simulink model "Drone_BBall_Developer"  (R2020a)
settings: Solver=FixedStepAuto  StartTime=0.0  StopTime=60  FixedStep=.001  RelTol=1e-3
values from neighbouring files (symbols this model uses):
  b = .25*m    (= 0.25)    [Run_Match.m]
  b_ball = .02*m_ball    (= 0.01)    [Run_Match.m]
  b_F_hook = 100    [Run_Match.m]
  b_F_hoop = m_ball * 50    (= 25)    [Run_Match.m]
  b_F_R = m * 20    (= 20)    [Run_Match.m]
  b_F_R_ball = m_ball * 10    (= 5)    [Run_Match.m]
  b_F_R_hook = m_hook * 100    (= 10)    [Run_Match.m]
  B_hook = r_hook^2*6*m_ball*g    (= 0.2943)    [Run_Match.m]
  b_hook = 0.05*m_hook    (= 0.005)    [Run_Match.m]
  b_tether = 1    [Run_Match.m]
  b_th = .1*J    (= 0.0192708333333)    [Run_Match.m]
  b_th_ball = .05*J_ball    (= 0.0009)    [Run_Match.m]
  b_x_net = 80*m_ball*g    (= 392.4)    [Run_Match.m]
  b_y_net = .4*m_ball*g    (= 1.962)    [Run_Match.m]
  drone = struct([])    [Run_Match.m]    (also in animate_drone_bball.m = [-r+w -r-w -r -r r r r+w r-w;             h    h  h  0 0 h  )
  g = 9.81    [Run_Match.m]
  J = 1/4*m*r^2 + 1/12*m*(2*(r+r_M_R))^2    (= 0.192708333333)    [Run_Match.m]
  J_ball = 2/5*m_ball*r_ball^2    (= 0.018)    [Run_Match.m]
  k_f = 4    [Run_Match.m]
  k_F_hook = 10000    [Run_Match.m]
  k_F_hoop = m_ball * 5000    (= 2500)    [Run_Match.m]
  k_F_R = m * 10000    (= 10000)    [Run_Match.m]
  k_F_R_ball = m_ball * 10000    (= 5000)    [Run_Match.m]
  k_F_R_hook = m_hook * 10000    (= 1000)    [Run_Match.m]
  k_tether = 40    [Run_Match.m]
  k_x_net = 200*m_ball*g    (= 981)    [Run_Match.m]
  k_y_net = .5*m_ball*g    (= 2.4525)    [Run_Match.m]
  L_tether = 1.0    (= 1)    [Run_Match.m]
  m = 1    [Run_Match.m]
  m_ball = .5    (= 0.5)    [Run_Match.m]
  m_hook = 0.1*m    (= 0.1)    [Run_Match.m]
  mu_f = .2    (= 0.2)    [Run_Match.m]
  mu_f_gnd = 0.5    [Run_Match.m]
  p_0 = [-5; 5]    [Run_Match.m]
  p_ball_0 = [0; r_ball]    [Run_Match.m]
  p_ball_dot_0 = [0; 12]    [Run_Match.m]
  p_emp = [0; -.4]    [Run_Match.m]
  p_emp_dot = [0; -5]    [Run_Match.m]
  p_hoop = [7.5 8; 8.5 8; -8.5 8; -7.5 8]'    [Run_Match.m]
  p_tether = [0; -0.259]    [Run_Match.m]
  r = 0.5    [Run_Match.m]    (also in animate_drone_bball.m = 0.475)
  r_ball = .3    (= 0.3)    [Run_Match.m]
  r_hook = 0.1    [Run_Match.m]
  r_M_R = 0.25*r    (= 0.125)    [Run_Match.m]
  T_0 = m*g    (= 9.81)    [Run_Match.m]
  T_max = 4*m*g    (= 39.24)    [Run_Match.m]
  T_tau = 0.1    [Run_Match.m]
undefined symbols (not defined in the file or in its folder): clock, M_max, sigbuilder_block, T_aux
libraries: dspswit3 x22, simulink x17, simulink_extras x3, dspmathops x2
(part 4 of 5)

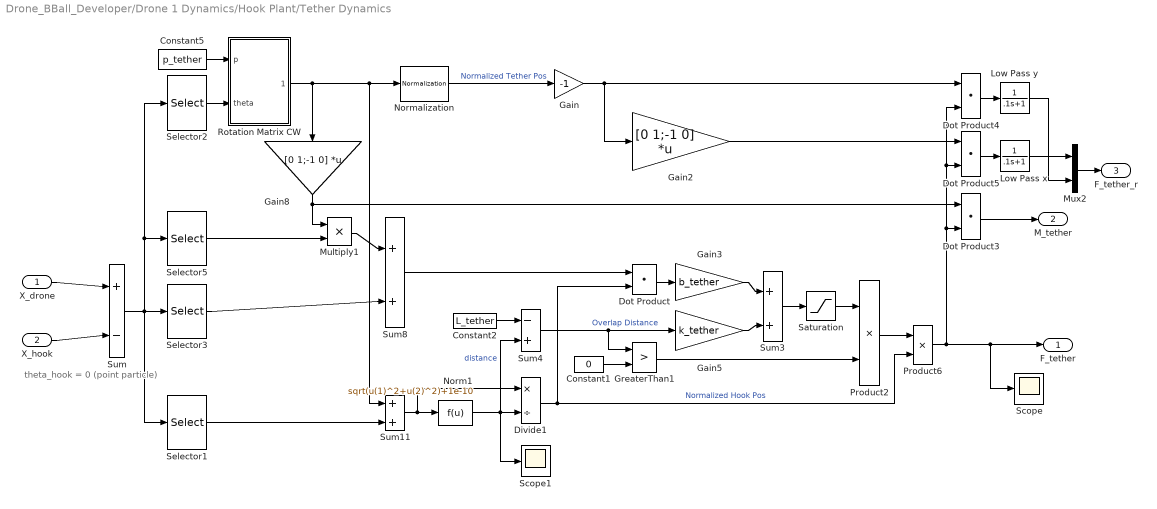
== system Drone_BBall_Developer/Drone 1 Dynamics/Hook Plant/Tether Dynamics ==
  note: theta_hook = 0
      | (point particle)
  X_drone : Inport
  X_hook : Inport  Port=2
  Constant1 : Constant  Value=0
  Constant2 : Constant  Value=L_tether
  Constant5 : Constant  Value=p_tether
  Divide1 : Product  Inputs=*/
  Dot Product{,3..5} (4 alike) : DotProduct  InputSameDT=on  OutDataTypeStr=Inherit: Inherit via internal rule
  Gain : Gain  Gain=-1
  Gain2 : Gain  Gain=[0 1;-1 0]  Multiplication=Matrix(K*u)
  Gain3 : Gain  Gain=b_tether
  Gain5 : Gain  Gain=k_tether
  Gain8 : Gain  Gain=[0 1;-1 0]  Multiplication=Matrix(K*u)
  GreaterThan1 : RelationalOperator  Operator=>  OutDataTypeStr=boolean  RndMeth=Simplest
  Low Pass x : TransferFcn  Denominator=[.1 1]
  Low Pass y : TransferFcn  Denominator=[.1 1]
  Multiply1 : Product
  Mux2 : Mux  Inputs=2
  Norm1 : Fcn  Expr=sqrt(u(1)^2+u(2)^2)+1e-10
  Normalization : dspmathops/Normalization  NormType=2-norm  Bias=1e-10  NormOver=Each column  Dimension=1  roundingMode=Floor  overflowMode=off  accumDataTypeStr=Inherit: Same as product output  accumLastDataTypeStr=Inherit: Same as product output  outputDataTypeStr=Inherit: Same as product output  outputMin=[]  outputMax=[]  outputLastDataTypeStr=Inherit: Same as product output
  Product2 : Product
  Product6 : Product
  Rotation Matrix CW : Subsystem
  Saturation : Saturate  UpperLimit=Inf  LowerLimit=0
  Scope : Scope
  Scope1 : Scope
  Selector1 : Selector  InputPortWidth=6  IndexOptions=Index vector (dialog)  Indices=[1 3]  OutputSizes=1
  Selector2 : Selector  InputPortWidth=6  IndexOptions=Index vector (dialog)  Indices=[5]  OutputSizes=1
  Selector3 : Selector  InputPortWidth=6  IndexOptions=Index vector (dialog)  Indices=[2 4]  OutputSizes=1
  Selector5 : Selector  InputPortWidth=6  IndexOptions=Index vector (dialog)  Indices=[6]  OutputSizes=1
  Sum : Sum  Inputs=+|-
  Sum11 : Sum
  Sum3 : Sum  Inputs=+|+
  Sum4 : Sum  Inputs=-+
  Sum8 : Sum  Inputs=+|||+
  F_tether : Outport  VectorParamsAs1DForOutWhenUnconnected=off
  M_tether : Outport  Port=2  VectorParamsAs1DForOutWhenUnconnected=off
  F_tether_r : Outport  Port=3  VectorParamsAs1DForOutWhenUnconnected=off
  wires:
  Constant1/1 -> GreaterThan1/2
  Sum11/1 -> Norm1/1, Divide1/1
  Sum4/1 -> Gain5/1, GreaterThan1/1  "Overlap Distance"
  X_drone/1 -> Sum/1
  Dot Product/1 -> Gain3/1
  Selector2/1 -> Rotation Matrix CW/2(theta)
  X_hook/1 -> Sum/2
  Gain5/1 -> Sum3/2
  Saturation/1 -> Product2/1
  Divide1/1 -> Product6/2, Dot Product/2  "Normalized Hook Pos"
  Norm1/1 -> Scope1/1, Sum4/2, Divide1/2  "distance"
  Sum8/1 -> Dot Product/1
  GreaterThan1/1 -> Product2/2
  Gain3/1 -> Sum3/1
  Sum3/1 -> Saturation/1
  Selector5/1 -> Multiply1/2
  Product2/1 -> Product6/1
  Constant2/1 -> Sum4/1
  Sum/1 -> Selector1/1, Selector2/1, Selector5/1, Selector3/1
  Constant5/1 -> Rotation Matrix CW/1(p)
  Rotation Matrix CW/1(R(theta)*p) -> Normalization/1, Sum11/1, Gain8/1
  Gain8/1 -> Dot Product3/1, Multiply1/1
  Multiply1/1 -> Sum8/1
  Selector3/1 -> Sum8/2
  Selector1/1 -> Sum11/2
  Dot Product3/1 -> M_tether/1
  Product6/1 -> Scope/1, F_tether/1, Dot Product5/2, Dot Product4/2, Dot Product3/2
  Normalization/1 -> Gain/1  "Normalized Tether Pos"
  Gain2/1 -> Dot Product5/1
  Dot Product5/1 -> Low Pass x/1
  Dot Product4/1 -> Low Pass y/1
  Mux2/1 -> F_tether_r/1
  Gain/1 -> Gain2/1, Dot Product4/1
  Low Pass x/1 -> Mux2/1
  Low Pass y/1 -> Mux2/2

== system Drone_BBall_Developer/Drone 1 Dynamics/Quadcopter Plant/Ceiling Reactions ==
  X : Inport
  Constant1 : Constant  Value=0
  Constant2 : Constant  Value=16-r
  Demux : Demux  Outputs=6
  Gain1 : Gain  Gain=r_M_R
  Gain10 : Gain  Gain=-k_f
  Gain12 : Gain  Gain=2
  Gain13 : Gain  Gain=r_M_R
  Gain4 : Gain  Gain=-b_F_R
  Gain6 : Gain  Gain=-k_F_R
  Gain8 : Gain  Gain=r
  Gain9 : Gain  Gain=r
  Less Than1 : RelationalOperator  Operator=<  OutDataTypeStr=boolean  RndMeth=Simplest
  Mux : Mux  Inputs=3
  Product5 : Product
  Product6 : Product  Inputs=3
  Product7 : Product
  Saturation : Saturate  UpperLimit=0  LowerLimit=-Inf
  Saturation1 : Saturate  UpperLimit=mu_f_gnd  LowerLimit=-mu_f_gnd
  Sin1 : Trigonometry
  Sin2 : Trigonometry  Operator=cos
  Sum3 : Sum  Inputs=|++
  Sum4 : Sum  Inputs=+-+
  Sum5 : Sum  Inputs=--|
  Sum6 : Sum  Inputs=++|
  Terminator : Terminator
  FM_R : Outport  VectorParamsAs1DForOutWhenUnconnected=off
  wires:
  Demux/2 -> Sum5/1
  Gain10/1 -> Saturation1/1
  Saturation1/1 -> Product6/1
  Saturation/1 -> Product5/2, Product6/2
  Demux/1 -> Terminator/1
  Product5/1 -> Product7/1, Mux/2
  Constant1/1 -> Less Than1/1
  Sum4/1 -> Less Than1/2, Gain6/1
  Demux/3 -> Sum4/3
  Product6/1 -> Mux/1, Gain8/1
  Demux/6 -> Gain9/1
  Gain4/1 -> Sum3/2
  Less Than1/1 -> Product6/3, Product5/1
  Sum3/1 -> Saturation/1
  Gain9/1 -> Sum5/2
  Sum5/1 -> Gain10/1
  Demux/4 -> Gain4/1
  Gain6/1 -> Sum3/1
  X/1 -> Demux/1
  Demux/5 -> Gain12/1
  Gain12/1 -> Sin2/1, Sin1/1
  Sin1/1 -> Gain13/1
  Gain13/1 -> Product7/2  "Moment arm of normal reaction force"
  Gain8/1 -> Sum6/1
  Sum6/1 -> Mux/3
  Product7/1 -> Sum6/2
  Mux/1 -> FM_R/1
  Sin2/1 -> Gain1/1
  Constant2/1 -> Sum4/2
  Gain1/1 -> Sum4/1

== system Drone_BBall_Developer/Drone 1 Dynamics/Quadcopter Plant/Ground Reactions ==
  X : Inport
  Constant1 : Constant  Value=0
  Constant2 : Constant  Value=r
  Demux : Demux  Outputs=6
  Gain1 : Gain  Gain=r_M_R
  Gain10 : Gain  Gain=-k_f
  Gain12 : Gain  Gain=2
  Gain13 : Gain  Gain=r_M_R
  Gain4 : Gain  Gain=-b_F_R
  Gain6 : Gain  Gain=-k_F_R
  Gain8 : Gain  Gain=-r
  Gain9 : Gain  Gain=r
  Less Than1 : RelationalOperator  Operator=>  OutDataTypeStr=boolean  RndMeth=Simplest
  Mux : Mux  Inputs=3
  Product5 : Product
  Product6 : Product  Inputs=3
  Product7 : Product
  Saturation : Saturate  UpperLimit=Inf  LowerLimit=0
  Saturation1 : Saturate  UpperLimit=mu_f_gnd  LowerLimit=-mu_f_gnd
  Sin1 : Trigonometry
  Sin2 : Trigonometry  Operator=cos
  Sum3 : Sum  Inputs=|++
  Sum4 : Sum  Inputs=+-+
  Sum5 : Sum  Inputs=+-|
  Sum6 : Sum  Inputs=+-|
  Terminator : Terminator
  FM_R : Outport  VectorParamsAs1DForOutWhenUnconnected=off
  wires:
  Demux/2 -> Sum5/1
  Gain10/1 -> Saturation1/1
  Saturation1/1 -> Product6/1
  Saturation/1 -> Product5/2, Product6/2
  Demux/1 -> Terminator/1
  Product5/1 -> Product7/1, Mux/2
  Constant1/1 -> Less Than1/1
  Sum4/1 -> Less Than1/2, Gain6/1
  Demux/3 -> Sum4/3
  Product6/1 -> Gain8/1, Mux/1
  Demux/6 -> Gain9/1
  Gain4/1 -> Sum3/2
  Less Than1/1 -> Product6/3, Product5/1
  Sum3/1 -> Saturation/1
  Gain9/1 -> Sum5/2
  Sum5/1 -> Gain10/1
  Demux/4 -> Gain4/1
  Gain6/1 -> Sum3/1
  X/1 -> Demux/1
  Demux/5 -> Gain12/1
  Gain12/1 -> Sin2/1, Sin1/1
  Sin1/1 -> Gain13/1
  Gain13/1 -> Product7/2  "Moment arm of normal reaction force"
  Gain8/1 -> Sum6/1
  Sum6/1 -> Mux/3
  Product7/1 -> Sum6/2
  Mux/1 -> FM_R/1
  Sin2/1 -> Gain1/1
  Constant2/1 -> Sum4/2
  Gain1/1 -> Sum4/1

== system Drone_BBall_Developer/Drone 1 Dynamics/Quadcopter Plant/Left Wall Reactions ==
  X : Inport
  Constant1 : Constant  Value=0
  Constant2 : Constant  Value=r-12
  Demux : Demux  Outputs=6
  Gain1 : Gain  Gain=r_M_R
  Gain10 : Gain  Gain=-k_f
  Gain12 : Gain  Gain=2
  Gain13 : Gain  Gain=r_M_R
  Gain4 : Gain  Gain=-b_F_R
  Gain6 : Gain  Gain=-k_F_R
  Gain8 : Gain  Gain=r
  Gain9 : Gain  Gain=r
  Less Than1 : RelationalOperator  Operator=<  OutDataTypeStr=boolean  RndMeth=Simplest
  Mux : Mux  Inputs=3
  Product5 : Product
  Product6 : Product  Inputs=3
  Product7 : Product
  Saturation : Saturate  UpperLimit=Inf  LowerLimit=0
  Saturation1 : Saturate  UpperLimit=mu_f_gnd  LowerLimit=-mu_f_gnd
  Sin1 : Trigonometry
  Sin2 : Trigonometry  Operator=cos
  Sum3 : Sum  Inputs=|++
  Sum4 : Sum  Inputs=--+
  Sum5 : Sum  Inputs=|++
  Sum6 : Sum  Inputs=++|
  Terminator : Terminator
  FM_R : Outport  VectorParamsAs1DForOutWhenUnconnected=off
  wires:
  Demux/4 -> Sum5/1
  Gain10/1 -> Saturation1/1
  Saturation1/1 -> Product6/3
  Saturation/1 -> Product5/1, Product6/2
  Product5/1 -> Product7/1, Mux/1
  Constant1/1 -> Less Than1/2
  Sum4/1 -> Less Than1/1, Gain6/1
  Demux/1 -> Sum4/3
  Product6/1 -> Mux/2, Gain8/1
  Demux/6 -> Gain9/1
  Gain4/1 -> Sum3/2
  Less Than1/1 -> Product5/2, Product6/1
  Sum3/1 -> Saturation/1
  Gain9/1 -> Sum5/2
  Sum5/1 -> Gain10/1
  Demux/2 -> Gain4/1
  Gain6/1 -> Sum3/1
  X/1 -> Demux/1
  Demux/5 -> Gain12/1
  Gain12/1 -> Sin2/1, Sin1/1
  Sin1/1 -> Gain13/1
  Gain13/1 -> Product7/2  "Moment arm of normal reaction force"
  Gain8/1 -> Sum6/1
  Sum6/1 -> Mux/3
  Product7/1 -> Sum6/2
  Mux/1 -> FM_R/1
  Sin2/1 -> Gain1/1
  Constant2/1 -> Sum4/2
  Gain1/1 -> Sum4/1
  Demux/3 -> Terminator/1

== system Drone_BBall_Developer/Drone 1 Dynamics/Quadcopter Plant/Linear Dynamics ==
  F : Inport
  Gain2 : Gain  Gain=1/m
  Gain5 : Gain  Gain=b
  Integrator4 : Integrator  InitialCondition=param.X_0([2 4])
  Integrator5 : Integrator  InitialCondition=param.X_0([1 3])
  Norm : Fcn  Expr=sqrt(u(1)^2+u(2)^2)
  Product4 : Product
  Sum3 : Sum  Inputs=+-
  p : Outport  VectorParamsAs1DForOutWhenUnconnected=off
  p_dot : Outport  Port=2  VectorParamsAs1DForOutWhenUnconnected=off
  wires:
  Integrator5/1 -> p/1
  F/1 -> Sum3/1
  Norm/1 -> Product4/2
  Integrator4/1 -> Integrator5/1, p_dot/1, Norm/1, Product4/1
  Sum3/1 -> Gain2/1
  Gain2/1 -> Integrator4/1
  Gain5/1 -> Sum3/2
  Product4/1 -> Gain5/1

== system Drone_BBall_Developer/Drone 1 Dynamics/Quadcopter Plant/Right Wall Reactions ==
  X : Inport
  Constant1 : Constant  Value=0
  Constant2 : Constant  Value=12-r
  Demux : Demux  Outputs=6
  Gain1 : Gain  Gain=r_M_R
  Gain10 : Gain  Gain=-k_f
  Gain12 : Gain  Gain=2
  Gain13 : Gain  Gain=r_M_R
  Gain4 : Gain  Gain=-b_F_R
  Gain6 : Gain  Gain=-k_F_R
  Gain8 : Gain  Gain=r
  Gain9 : Gain  Gain=r
  Less Than1 : RelationalOperator  Operator=>  OutDataTypeStr=boolean  RndMeth=Simplest
  Mux : Mux  Inputs=3
  Product5 : Product
  Product6 : Product  Inputs=3
  Product7 : Product
  Saturation : Saturate  UpperLimit=0  LowerLimit=-Inf
  Saturation1 : Saturate  UpperLimit=mu_f_gnd  LowerLimit=-mu_f_gnd
  Sin1 : Trigonometry
  Sin2 : Trigonometry  Operator=cos
  Sum3 : Sum  Inputs=|++
  Sum4 : Sum  Inputs=--+
  Sum5 : Sum  Inputs=|-+
  Sum6 : Sum  Inputs=+-|
  Terminator : Terminator
  FM_R : Outport  VectorParamsAs1DForOutWhenUnconnected=off
  wires:
  Demux/4 -> Sum5/1
  Gain10/1 -> Saturation1/1
  Saturation1/1 -> Product6/3
  Saturation/1 -> Product5/1, Product6/2
  Product5/1 -> Product7/1, Mux/1
  Constant1/1 -> Less Than1/2
  Sum4/1 -> Less Than1/1, Gain6/1
  Demux/1 -> Sum4/3
  Product6/1 -> Mux/2, Gain8/1
  Demux/6 -> Gain9/1
  Gain4/1 -> Sum3/2
  Less Than1/1 -> Product5/2, Product6/1
  Sum3/1 -> Saturation/1
  Gain9/1 -> Sum5/2
  Sum5/1 -> Gain10/1
  Demux/2 -> Gain4/1
  Gain6/1 -> Sum3/1
  X/1 -> Demux/1
  Demux/5 -> Gain12/1
  Gain12/1 -> Sin2/1, Sin1/1
  Sin1/1 -> Gain13/1
  Gain13/1 -> Product7/2  "Moment arm of normal reaction force"
  Gain8/1 -> Sum6/1
  Sum6/1 -> Mux/3
  Product7/1 -> Sum6/2
  Mux/1 -> FM_R/1
  Sin2/1 -> Gain1/1
  Constant2/1 -> Sum4/2
  Gain1/1 -> Sum4/1
  Demux/3 -> Terminator/1

== system Drone_BBall_Developer/Drone 1 Dynamics/Quadcopter Plant/Rotational Dynamics ==
  M : Inport
  Fcn1 : Fcn  Expr=u*abs(u)
  Gain : Gain  Gain=b_th
  Gain1 : Gain  Gain=1/J
  Integrator : Integrator  InitialCondition=param.X_0(6)
  Integrator1 : Integrator  InitialCondition=param.X_0(5)
  Sum2 : Sum  Inputs=|+-
  Wrap Angle : Subsystem
  theta : Outport  VectorParamsAs1DForOutWhenUnconnected=off
  theta_dot : Outport  Port=2  VectorParamsAs1DForOutWhenUnconnected=off
  wires:
  Integrator1/1 -> Wrap Angle/1(raw)
  Integrator/1 -> Integrator1/1, Fcn1/1, theta_dot/1
  Gain1/1 -> Integrator/1
  Wrap Angle/1(wrap) -> theta/1
  Fcn1/1 -> Gain/1
  M/1 -> Sum2/1
  Gain/1 -> Sum2/2
  Sum2/1 -> Gain1/1

== system Drone_BBall_Developer/Drone 1 Dynamics/Quadcopter Plant/Thrust Dynamics ==
  T_d : Inport
  Gain : Gain  Gain=1/T_tau
  Integrator : Integrator  InitialCondition=T_0/2
  Sum : Sum  Inputs=|+-
  Thrust Limit : Saturate  UpperLimit=T_max  LowerLimit=0
  T : Outport  VectorParamsAs1DForOutWhenUnconnected=off
  wires:
  Gain/1 -> Integrator/1
  Sum/1 -> Gain/1
  Thrust Limit/1 -> Sum/1
  T_d/1 -> Thrust Limit/1
  Integrator/1 -> T/1, Sum/2

== system Drone_BBall_Developer/Drone 1 Dynamics/Quadcopter Plant/Thrust Dynamics L ==
  T_d : Inport
  Gain : Gain  Gain=1/T_tau
  Integrator : Integrator  InitialCondition=T_0/2
  Sum : Sum  Inputs=|+-
  Thrust Limit : Saturate  UpperLimit=T_max  LowerLimit=0
  T : Outport  VectorParamsAs1DForOutWhenUnconnected=off
  wires:
  Gain/1 -> Integrator/1
  Sum/1 -> Gain/1
  Thrust Limit/1 -> Sum/1
  T_d/1 -> Thrust Limit/1
  Integrator/1 -> T/1, Sum/2

== system Drone_BBall_Developer/Drone 1 Dynamics/Quadcopter Plant/Thrust Resultants ==
  T_L : Inport
  T_R : Inport  Port=2
  Theta : Inport  Port=3
  Gain : Gain  Gain=r
  Mux : Mux  Inputs=3
  Product : Product
  Product1 : Product
  Sin : Trigonometry
  Sin1 : Trigonometry  Operator=cos
  Sum : Sum  Inputs=|++
  Sum1 : Sum  Inputs=+-|
  "FM " : Outport  VectorParamsAs1DForOutWhenUnconnected=off
  wires:
  T_L/1 -> Sum/1, Sum1/1
  T_R/1 -> Sum/2, Sum1/2
  Gain/1 -> Mux/3  "M"
  Sum1/1 -> Gain/1
  Sum/1 -> Product1/1, Product/1
  Sin1/1 -> Product1/2
  Theta/1 -> Sin/1, Sin1/1
  Product/1 -> Mux/1  "F_x"
  Sin/1 -> Product/2
  Mux/1 -> "FM "/1
  Product1/1 -> Mux/2  "F_y"

== system Drone_BBall_Developer/Drone 2 Dynamics/Hook Plant/Ground Reactions ==
  X : Inport
  Constant1 : Constant  Value=0
  Demux : Demux  Outputs=6
  Gain : Gain  Gain=-k_F_R_hook
  Gain4 : Gain  Gain=-b_F_R_hook
  Gain6 : Gain  Gain=-k_f
  Less Than1 : RelationalOperator  Operator=>  OutDataTypeStr=boolean  RndMeth=Simplest
  Mux : Mux  Inputs=2
  Product2 : Product
  Product5 : Product  Inputs=3
  Saturation : Saturate  UpperLimit=Inf  LowerLimit=0
  Saturation1 : Saturate  UpperLimit=mu_f  LowerLimit=-mu_f
  Sum1 : Sum  Inputs=|++
  Terminator : Terminator
  Terminator1 : Terminator
  Terminator2 : Terminator
  F_R : Outport  VectorParamsAs1DForOutWhenUnconnected=off
  wires:
  Gain6/1 -> Saturation1/1
  Saturation1/1 -> Product5/1
  Saturation/1 -> Product2/2, Product5/2
  Demux/1 -> Terminator/1
  Mux/1 -> F_R/1
  Product2/1 -> Mux/2
  Demux/5 -> Terminator1/1
  Constant1/1 -> Less Than1/1
  Demux/3 -> Gain/1, Less Than1/2
  Product5/1 -> Mux/1
  Gain4/1 -> Sum1/2
  Less Than1/1 -> Product5/3, Product2/1
  Sum1/1 -> Saturation/1
  Demux/2 -> Gain6/1
  Demux/4 -> Gain4/1
  Gain/1 -> Sum1/1
  X/1 -> Demux/1
  Demux/6 -> Terminator2/1

== system Drone_BBall_Developer/Drone 2 Dynamics/Hook Plant/Hook Dynamics ==
  X_hook : Inport
  X_ball : Inport  Port=2
  mag_on : Inport  Port=3
  Constant : Constant  Value=0
  Constant1 : Constant  Value=r_ball
  Constant2 : Constant  Value=r_ball
  Constant3 : Constant  Value=r_hook
  Divide1 : Product  Inputs=**/
  Divide2 : Product  Inputs=*/
  Dot Product : DotProduct  InputSameDT=on  OutDataTypeStr=Inherit: Inherit via internal rule
  Dot Product1 : DotProduct  InputSameDT=on  OutDataTypeStr=Inherit: Inherit via internal rule
  Gain : Gain  Gain=r_ball
  Gain1 : Gain  Gain=-k_f
  Gain2 : Gain  Gain=b_F_hook
  Gain3 : Gain  Gain=k_F_hook
  Gain6 : Gain  Gain=B_hook
  Gain7 : Gain  Gain=[0 1;-1 0]  Multiplication=Matrix(K*u)
  GreaterThan : RelationalOperator  Operator=>  OutDataTypeStr=boolean  RndMeth=Simplest
  Norm : Fcn  Expr=sqrt(u(1)^2+u(2)^2)+1e-10
  Product : Product  Inputs=3
  Product{1..5} (5 alike) : Product
  Saturation : Saturate  UpperLimit=0  LowerLimit=-Inf
  Saturation1 : Saturate  UpperLimit=mu_f  LowerLimit=-mu_f
  Selector : Selector  InputPortWidth=6  IndexOptions=Index vector (dialog)  Indices=[1 3]  OutputSizes=1
  Selector1 : Selector  InputPortWidth=6  IndexOptions=Index vector (dialog)  Indices=[6]  OutputSizes=1
  Selector2 : Selector  InputPortWidth=6  IndexOptions=Index vector (dialog)  Indices=[2 4]  OutputSizes=1
  Square : Math  Operator=square  SignedPower=on  SaturateOnIntegerOverflow=on
  Sum : Sum  Inputs=+-
  Sum1 : Sum  Inputs=+||+|||+
  Sum2 : Sum  Inputs=+|+
  Sum3 : Sum  Inputs=-|+
  Sum4 : Sum  Inputs=++|
  Sum5 : Sum  Inputs=+-+
  F_ball : Outport  VectorParamsAs1DForOutWhenUnconnected=off
  M_ball : Outport  Port=2  VectorParamsAs1DForOutWhenUnconnected=off
  wires:
  Gain/1 -> M_ball/1
  mag_on/1 -> Divide1/2
  X_hook/1 -> Sum/1
  X_ball/1 -> Sum/2
  Sum/1 -> Selector1/1, Selector2/1, Selector/1
  Selector/1 -> Divide2/1, Norm/1
  Sum3/1 -> Product1/2, GreaterThan/2  "Overlap Distance"
  Constant/1 -> GreaterThan/1
  GreaterThan/1 -> Product1/1, Product3/2
  Product3/1 -> Gain2/1
  Sum1/1 -> F_ball/1
  Dot Product1/1 -> Gain1/1
  Gain2/1 -> Sum2/1
  Gain3/1 -> Sum2/2
  Product5/1 -> Product2/1, Gain/1
  Divide1/1 -> Gain6/1
  Gain6/1 -> Sum1/3  "Magnetic Force"
  Norm/1 -> Sum5/1, Divide2/2, Product/2, Sum3/2  "radius"
  Constant1/1 -> Sum3/1
  Divide2/1 -> Divide1/1, Product4/2, Gain7/1, Dot Product/2  "Normalized Pos Vector"
  Dot Product/1 -> Product3/1
  Product1/1 -> Gain3/1
  Square/1 -> Divide1/3  "Squared Distance"
  Gain7/1 -> Product/3, Product2/2, Dot Product1/2  "Tangent Vector"
  Product/1 -> Sum4/2
  Selector2/1 -> Sum4/1
  Sum4/1 -> Dot Product/1, Dot Product1/1
  Selector1/1 -> Product/1  "theta_dot"
  Gain1/1 -> Saturation1/1
  Product4/1 -> Sum1/2  "Normal Force"
  Product2/1 -> Sum1/1  "Friction Force"
  Saturation/1 -> Product5/2, Product4/1
  Sum2/1 -> Saturation/1
  Saturation1/1 -> Product5/1
  Constant2/1 -> Sum5/2
  Constant3/1 -> Sum5/3
  Sum5/1 -> Square/1  "Magnet Distance"

== system Drone_BBall_Developer/Drone 2 Dynamics/Hook Plant/Linear Dynamics ==
  F : Inport
  Gain : Gain  Gain=1/m_hook
  Gain1 : Gain  Gain=b_hook
  Integrator : Integrator  InitialCondition=param.X_0([1 3])+p_tether+[0;-L_tether]
  Integrator1 : Integrator  InitialCondition=param.X_0([2 4])
  Norm : Fcn  Expr=sqrt(u(1)^2+u(2)^2)
  Product : Product
  Sum3 : Sum  Inputs=+-
  p : Outport  VectorParamsAs1DForOutWhenUnconnected=off
  p_dot : Outport  Port=2  VectorParamsAs1DForOutWhenUnconnected=off
  wires:
  Gain1/1 -> Sum3/2
  Integrator1/1 -> Integrator/1, Norm/1, Product/1, p_dot/1
  Norm/1 -> Product/2
  Product/1 -> Gain1/1
  F/1 -> Sum3/1
  Sum3/1 -> Gain/1
  Gain/1 -> Integrator1/1
  Integrator/1 -> p/1

== system Drone_BBall_Developer/Drone 2 Dynamics/Hook Plant/Tether Dynamics ==
  note: theta_hook = 0
      | (point particle)
  X_drone : Inport
  X_hook : Inport  Port=2
  Constant1 : Constant  Value=0
  Constant2 : Constant  Value=L_tether
  Constant5 : Constant  Value=p_tether
  Divide1 : Product  Inputs=*/
  Dot Product{,3..5} (4 alike) : DotProduct  InputSameDT=on  OutDataTypeStr=Inherit: Inherit via internal rule
  Gain : Gain  Gain=-1
  Gain2 : Gain  Gain=[0 1;-1 0]  Multiplication=Matrix(K*u)
  Gain3 : Gain  Gain=b_tether
  Gain5 : Gain  Gain=k_tether
  Gain8 : Gain  Gain=[0 1;-1 0]  Multiplication=Matrix(K*u)
  GreaterThan1 : RelationalOperator  Operator=>  OutDataTypeStr=boolean  RndMeth=Simplest
  Multiply1 : Product
  Mux2 : Mux  Inputs=2
  Norm1 : Fcn  Expr=sqrt(u(1)^2+u(2)^2)+1e-10
  Normalization : dspmathops/Normalization  NormType=2-norm  Bias=1e-10  NormOver=Each column  Dimension=1  roundingMode=Floor  overflowMode=off  accumDataTypeStr=Inherit: Same as product output  accumLastDataTypeStr=Inherit: Same as product output  outputDataTypeStr=Inherit: Same as product output  outputMin=[]  outputMax=[]  outputLastDataTypeStr=Inherit: Same as product output
  Product2 : Product
  Product6 : Product
  Rotation Matrix CW : Subsystem
  Saturation : Saturate  UpperLimit=Inf  LowerLimit=0
  Selector1 : Selector  InputPortWidth=6  IndexOptions=Index vector (dialog)  Indices=[1 3]  OutputSizes=1
  Selector2 : Selector  InputPortWidth=6  IndexOptions=Index vector (dialog)  Indices=[5]  OutputSizes=1
  Selector3 : Selector  InputPortWidth=6  IndexOptions=Index vector (dialog)  Indices=[2 4]  OutputSizes=1
  Selector5 : Selector  InputPortWidth=6  IndexOptions=Index vector (dialog)  Indices=[6]  OutputSizes=1
  Sum : Sum  Inputs=+|-
  Sum11 : Sum
  Sum3 : Sum  Inputs=+|+
  Sum4 : Sum  Inputs=-+
  Sum8 : Sum  Inputs=+|||+
  F_tether : Outport  VectorParamsAs1DForOutWhenUnconnected=off
  M_tether : Outport  Port=2  VectorParamsAs1DForOutWhenUnconnected=off
  F_tether_r : Outport  Port=3  VectorParamsAs1DForOutWhenUnconnected=off
  wires:
  Constant1/1 -> GreaterThan1/2
  Sum11/1 -> Norm1/1, Divide1/1
  Sum4/1 -> Gain5/1, GreaterThan1/1  "Overlap Distance"
  X_drone/1 -> Sum/1
  Dot Product/1 -> Gain3/1
  Selector2/1 -> Rotation Matrix CW/2(theta)
  X_hook/1 -> Sum/2
  Gain5/1 -> Sum3/2
  Saturation/1 -> Product2/1
  Divide1/1 -> Product6/2, Dot Product/2  "Normalized Hook Pos"
  Norm1/1 -> Sum4/2, Divide1/2  "distance"
  Sum8/1 -> Dot Product/1
  GreaterThan1/1 -> Product2/2
  Gain3/1 -> Sum3/1
  Sum3/1 -> Saturation/1
  Selector5/1 -> Multiply1/2
  Product2/1 -> Product6/1
  Constant2/1 -> Sum4/1
  Sum/1 -> Selector1/1, Selector2/1, Selector5/1, Selector3/1
  Constant5/1 -> Rotation Matrix CW/1(p)
  Rotation Matrix CW/1(R(theta)*p) -> Normalization/1, Sum11/1, Gain8/1
  Gain8/1 -> Dot Product3/1, Multiply1/1
  Multiply1/1 -> Sum8/1
  Selector3/1 -> Sum8/2
  Selector1/1 -> Sum11/2
  Dot Product3/1 -> M_tether/1
  Product6/1 -> F_tether/1, Dot Product5/2, Dot Product4/2, Dot Product3/2
  Normalization/1 -> Gain/1  "Normalized Tether Pos"
  Gain2/1 -> Dot Product5/1
  Dot Product5/1 -> Mux2/1
  Dot Product4/1 -> Mux2/2
  Mux2/1 -> F_tether_r/1
  Gain/1 -> Gain2/1, Dot Product4/1

== system Drone_BBall_Developer/Drone 2 Dynamics/Quadcopter Plant/Ceiling Reactions ==
  X : Inport
  Constant1 : Constant  Value=0
  Constant2 : Constant  Value=16-r
  Demux : Demux  Outputs=6
  Gain1 : Gain  Gain=r_M_R
  Gain10 : Gain  Gain=-k_f
  Gain12 : Gain  Gain=2
  Gain13 : Gain  Gain=r_M_R
  Gain4 : Gain  Gain=-b_F_R
  Gain6 : Gain  Gain=-k_F_R
  Gain8 : Gain  Gain=r
  Gain9 : Gain  Gain=r
  Less Than1 : RelationalOperator  Operator=<  OutDataTypeStr=boolean  RndMeth=Simplest
  Mux : Mux  Inputs=3
  Product5 : Product
  Product6 : Product  Inputs=3
  Product7 : Product
  Saturation : Saturate  UpperLimit=0  LowerLimit=-Inf
  Saturation1 : Saturate  UpperLimit=mu_f_gnd  LowerLimit=-mu_f_gnd
  Sin1 : Trigonometry
  Sin2 : Trigonometry  Operator=cos
  Sum3 : Sum  Inputs=|++
  Sum4 : Sum  Inputs=+-+
  Sum5 : Sum  Inputs=--|
  Sum6 : Sum  Inputs=++|
  Terminator : Terminator
  FM_R : Outport  VectorParamsAs1DForOutWhenUnconnected=off
  wires:
  Demux/2 -> Sum5/1
  Gain10/1 -> Saturation1/1
  Saturation1/1 -> Product6/1
  Saturation/1 -> Product5/2, Product6/2
  Demux/1 -> Terminator/1
  Product5/1 -> Product7/1, Mux/2
  Constant1/1 -> Less Than1/1
  Sum4/1 -> Less Than1/2, Gain6/1
  Demux/3 -> Sum4/3
  Product6/1 -> Mux/1, Gain8/1
  Demux/6 -> Gain9/1
  Gain4/1 -> Sum3/2
  Less Than1/1 -> Product6/3, Product5/1
  Sum3/1 -> Saturation/1
  Gain9/1 -> Sum5/2
  Sum5/1 -> Gain10/1
  Demux/4 -> Gain4/1
  Gain6/1 -> Sum3/1
  X/1 -> Demux/1
  Demux/5 -> Gain12/1
  Gain12/1 -> Sin2/1, Sin1/1
  Sin1/1 -> Gain13/1
  Gain13/1 -> Product7/2  "Moment arm of normal reaction force"
  Gain8/1 -> Sum6/1
  Sum6/1 -> Mux/3
  Product7/1 -> Sum6/2
  Mux/1 -> FM_R/1
  Sin2/1 -> Gain1/1
  Constant2/1 -> Sum4/2
  Gain1/1 -> Sum4/1

== system Drone_BBall_Developer/Drone 2 Dynamics/Quadcopter Plant/Ground Reactions ==
  X : Inport
  Constant1 : Constant  Value=0
  Constant2 : Constant  Value=r
  Demux : Demux  Outputs=6
  Gain1 : Gain  Gain=r_M_R
  Gain10 : Gain  Gain=-k_f
  Gain12 : Gain  Gain=2
  Gain13 : Gain  Gain=r_M_R
  Gain4 : Gain  Gain=-b_F_R
  Gain6 : Gain  Gain=-k_F_R
  Gain8 : Gain  Gain=-r
  Gain9 : Gain  Gain=r
  Less Than1 : RelationalOperator  Operator=>  OutDataTypeStr=boolean  RndMeth=Simplest
  Mux : Mux  Inputs=3
  Product5 : Product
  Product6 : Product  Inputs=3
  Product7 : Product
  Saturation : Saturate  UpperLimit=Inf  LowerLimit=0
  Saturation1 : Saturate  UpperLimit=mu_f_gnd  LowerLimit=-mu_f_gnd
  Sin1 : Trigonometry
  Sin2 : Trigonometry  Operator=cos
  Sum3 : Sum  Inputs=|++
  Sum4 : Sum  Inputs=+-+
  Sum5 : Sum  Inputs=+-|
  Sum6 : Sum  Inputs=+-|
  Terminator : Terminator
  FM_R : Outport  VectorParamsAs1DForOutWhenUnconnected=off
  wires:
  Demux/2 -> Sum5/1
  Gain10/1 -> Saturation1/1
  Saturation1/1 -> Product6/1
  Saturation/1 -> Product5/2, Product6/2
  Demux/1 -> Terminator/1
  Product5/1 -> Product7/1, Mux/2
  Constant1/1 -> Less Than1/1
  Sum4/1 -> Less Than1/2, Gain6/1
  Demux/3 -> Sum4/3
  Product6/1 -> Gain8/1, Mux/1
  Demux/6 -> Gain9/1
  Gain4/1 -> Sum3/2
  Less Than1/1 -> Product6/3, Product5/1
  Sum3/1 -> Saturation/1
  Gain9/1 -> Sum5/2
  Sum5/1 -> Gain10/1
  Demux/4 -> Gain4/1
  Gain6/1 -> Sum3/1
  X/1 -> Demux/1
  Demux/5 -> Gain12/1
  Gain12/1 -> Sin2/1, Sin1/1
  Sin1/1 -> Gain13/1
  Gain13/1 -> Product7/2  "Moment arm of normal reaction force"
  Gain8/1 -> Sum6/1
  Sum6/1 -> Mux/3
  Product7/1 -> Sum6/2
  Mux/1 -> FM_R/1
  Sin2/1 -> Gain1/1
  Constant2/1 -> Sum4/2
  Gain1/1 -> Sum4/1

== system Drone_BBall_Developer/Drone 2 Dynamics/Quadcopter Plant/Left Wall Reactions ==
  X : Inport
  Constant1 : Constant  Value=0
  Constant2 : Constant  Value=r-12
  Demux : Demux  Outputs=6
  Gain1 : Gain  Gain=r_M_R
  Gain10 : Gain  Gain=-k_f
  Gain12 : Gain  Gain=2
  Gain13 : Gain  Gain=r_M_R
  Gain4 : Gain  Gain=-b_F_R
  Gain6 : Gain  Gain=-k_F_R
  Gain8 : Gain  Gain=r
  Gain9 : Gain  Gain=r
  Less Than1 : RelationalOperator  Operator=<  OutDataTypeStr=boolean  RndMeth=Simplest
  Mux : Mux  Inputs=3
  Product5 : Product
  Product6 : Product  Inputs=3
  Product7 : Product
  Saturation : Saturate  UpperLimit=Inf  LowerLimit=0
  Saturation1 : Saturate  UpperLimit=mu_f_gnd  LowerLimit=-mu_f_gnd
  Sin1 : Trigonometry
  Sin2 : Trigonometry  Operator=cos
  Sum3 : Sum  Inputs=|++
  Sum4 : Sum  Inputs=--+
  Sum5 : Sum  Inputs=|++
  Sum6 : Sum  Inputs=++|
  Terminator : Terminator
  FM_R : Outport  VectorParamsAs1DForOutWhenUnconnected=off
  wires:
  Demux/4 -> Sum5/1
  Gain10/1 -> Saturation1/1
  Saturation1/1 -> Product6/3
  Saturation/1 -> Product5/1, Product6/2
  Product5/1 -> Product7/1, Mux/1
  Constant1/1 -> Less Than1/2
  Sum4/1 -> Less Than1/1, Gain6/1
  Demux/1 -> Sum4/3
  Product6/1 -> Mux/2, Gain8/1
  Demux/6 -> Gain9/1
  Gain4/1 -> Sum3/2
  Less Than1/1 -> Product5/2, Product6/1
  Sum3/1 -> Saturation/1
  Gain9/1 -> Sum5/2
  Sum5/1 -> Gain10/1
  Demux/2 -> Gain4/1
  Gain6/1 -> Sum3/1
  X/1 -> Demux/1
  Demux/5 -> Gain12/1
  Gain12/1 -> Sin2/1, Sin1/1
  Sin1/1 -> Gain13/1
  Gain13/1 -> Product7/2  "Moment arm of normal reaction force"
  Gain8/1 -> Sum6/1
  Sum6/1 -> Mux/3
  Product7/1 -> Sum6/2
  Mux/1 -> FM_R/1
  Sin2/1 -> Gain1/1
  Constant2/1 -> Sum4/2
  Gain1/1 -> Sum4/1
  Demux/3 -> Terminator/1

== system Drone_BBall_Developer/Drone 2 Dynamics/Quadcopter Plant/Linear Dynamics ==
  F : Inport
  Gain2 : Gain  Gain=1/m
  Gain5 : Gain  Gain=b
  Integrator4 : Integrator  InitialCondition=param.X_0([2 4])
  Integrator5 : Integrator  InitialCondition=param.X_0([1 3])
  Norm : Fcn  Expr=sqrt(u(1)^2+u(2)^2)
  Product4 : Product
  Sum3 : Sum  Inputs=+-
  p : Outport  VectorParamsAs1DForOutWhenUnconnected=off
  p_dot : Outport  Port=2  VectorParamsAs1DForOutWhenUnconnected=off
  wires:
  Integrator5/1 -> p/1
  F/1 -> Sum3/1
  Norm/1 -> Product4/2
  Integrator4/1 -> Integrator5/1, Norm/1, Product4/1, p_dot/1
  Sum3/1 -> Gain2/1
  Gain2/1 -> Integrator4/1
  Gain5/1 -> Sum3/2
  Product4/1 -> Gain5/1

== system Drone_BBall_Developer/Drone 2 Dynamics/Quadcopter Plant/Right Wall Reactions ==
  X : Inport
  Constant1 : Constant  Value=0
  Constant2 : Constant  Value=12-r
  Demux : Demux  Outputs=6
  Gain1 : Gain  Gain=r_M_R
  Gain10 : Gain  Gain=-k_f
  Gain12 : Gain  Gain=2
  Gain13 : Gain  Gain=r_M_R
  Gain4 : Gain  Gain=-b_F_R
  Gain6 : Gain  Gain=-k_F_R
  Gain8 : Gain  Gain=r
  Gain9 : Gain  Gain=r
  Less Than1 : RelationalOperator  Operator=>  OutDataTypeStr=boolean  RndMeth=Simplest
  Mux : Mux  Inputs=3
  Product5 : Product
  Product6 : Product  Inputs=3
  Product7 : Product
  Saturation : Saturate  UpperLimit=0  LowerLimit=-Inf
  Saturation1 : Saturate  UpperLimit=mu_f_gnd  LowerLimit=-mu_f_gnd
  Sin1 : Trigonometry
  Sin2 : Trigonometry  Operator=cos
  Sum3 : Sum  Inputs=|++
  Sum4 : Sum  Inputs=--+
  Sum5 : Sum  Inputs=|-+
  Sum6 : Sum  Inputs=+-|
  Terminator : Terminator
  FM_R : Outport  VectorParamsAs1DForOutWhenUnconnected=off
  wires:
  Demux/4 -> Sum5/1
  Gain10/1 -> Saturation1/1
  Saturation1/1 -> Product6/3
  Saturation/1 -> Product5/1, Product6/2
  Product5/1 -> Product7/1, Mux/1
  Constant1/1 -> Less Than1/2
  Sum4/1 -> Less Than1/1, Gain6/1
  Demux/1 -> Sum4/3
  Product6/1 -> Mux/2, Gain8/1
  Demux/6 -> Gain9/1
  Gain4/1 -> Sum3/2
  Less Than1/1 -> Product5/2, Product6/1
  Sum3/1 -> Saturation/1
  Gain9/1 -> Sum5/2
  Sum5/1 -> Gain10/1
  Demux/2 -> Gain4/1
  Gain6/1 -> Sum3/1
  X/1 -> Demux/1
  Demux/5 -> Gain12/1
  Gain12/1 -> Sin2/1, Sin1/1
  Sin1/1 -> Gain13/1
  Gain13/1 -> Product7/2  "Moment arm of normal reaction force"
  Gain8/1 -> Sum6/1
  Sum6/1 -> Mux/3
  Product7/1 -> Sum6/2
  Mux/1 -> FM_R/1
  Sin2/1 -> Gain1/1
  Constant2/1 -> Sum4/2
  Gain1/1 -> Sum4/1
  Demux/3 -> Terminator/1

== system Drone_BBall_Developer/Drone 2 Dynamics/Quadcopter Plant/Rotational Dynamics ==
  M : Inport
  Fcn1 : Fcn  Expr=u*abs(u)
  Gain : Gain  Gain=b_th
  Gain1 : Gain  Gain=1/J
  Integrator : Integrator  InitialCondition=param.X_0(6)
  Integrator1 : Integrator  InitialCondition=param.X_0(5)
  Sum2 : Sum  Inputs=|+-
  Wrap Angle : Subsystem
  theta : Outport  VectorParamsAs1DForOutWhenUnconnected=off
  theta_dot : Outport  Port=2  VectorParamsAs1DForOutWhenUnconnected=off
  wires:
  Integrator1/1 -> Wrap Angle/1(raw)
  Integrator/1 -> Integrator1/1, Fcn1/1, theta_dot/1
  Gain1/1 -> Integrator/1
  Wrap Angle/1(wrap) -> theta/1
  Fcn1/1 -> Gain/1
  M/1 -> Sum2/1
  Gain/1 -> Sum2/2
  Sum2/1 -> Gain1/1

== system Drone_BBall_Developer/Drone 2 Dynamics/Quadcopter Plant/Thrust Dynamics ==
  T_d : Inport
  Gain : Gain  Gain=1/T_tau
  Integrator : Integrator  InitialCondition=T_0/2
  Sum : Sum  Inputs=|+-
  Thrust Limit : Saturate  UpperLimit=T_max  LowerLimit=0
  T : Outport  VectorParamsAs1DForOutWhenUnconnected=off
  wires:
  Gain/1 -> Integrator/1
  Sum/1 -> Gain/1
  Thrust Limit/1 -> Sum/1
  T_d/1 -> Thrust Limit/1
  Integrator/1 -> T/1, Sum/2

== system Drone_BBall_Developer/Drone 2 Dynamics/Quadcopter Plant/Thrust Dynamics L ==
  T_d : Inport
  Gain : Gain  Gain=1/T_tau
  Integrator : Integrator  InitialCondition=T_0/2
  Sum : Sum  Inputs=|+-
  Thrust Limit : Saturate  UpperLimit=T_max  LowerLimit=0
  T : Outport  VectorParamsAs1DForOutWhenUnconnected=off
  wires:
  Gain/1 -> Integrator/1
  Sum/1 -> Gain/1
  Thrust Limit/1 -> Sum/1
  T_d/1 -> Thrust Limit/1
  Integrator/1 -> T/1, Sum/2

== system Drone_BBall_Developer/Drone 2 Dynamics/Quadcopter Plant/Thrust Resultants ==
  T_L : Inport
  T_R : Inport  Port=2
  Theta : Inport  Port=3
  Gain : Gain  Gain=r
  Mux : Mux  Inputs=3
  Product : Product
  Product1 : Product
  Sin : Trigonometry
  Sin1 : Trigonometry  Operator=cos
  Sum : Sum  Inputs=|++
  Sum1 : Sum  Inputs=+-|
  "FM " : Outport  VectorParamsAs1DForOutWhenUnconnected=off
  wires:
  T_L/1 -> Sum/1, Sum1/1
  T_R/1 -> Sum/2, Sum1/2
  Gain/1 -> Mux/3  "M"
  Sum1/1 -> Gain/1
  Product1/1 -> Mux/2  "F_y"
  Sin1/1 -> Product1/2
  Theta/1 -> Sin/1, Sin1/1
  Product/1 -> Mux/1  "F_x"
  Sin/1 -> Product/2
  Sum/1 -> Product1/1, Product/1
  Mux/1 -> "FM "/1

== system Drone_BBall_Developer/EMP Mechanics//Dynamics/EMP Dynamics 1/Rotation Matrx ==
  p : Inport
  theta : Inport  Port=2
  Cos : Trigonometry  Operator=cos
  Demux : Demux  Outputs=2
  Demux1 : Demux  Outputs=2
  Mux3 : Mux  Inputs=2
  Product : Product
  Product1 : Product
  Sin : Trigonometry
  Sum1 : Sum
  Sum2 : Sum  Inputs=+-
  R(theta)*p : Outport  VectorParamsAs1DForOutWhenUnconnected=off
  wires:
  p/1 -> Product/2, Product1/2
  Sum2/1 -> Mux3/2
  Sin/1 -> Product1/1
  theta/1 -> Cos/1, Sin/1
  Cos/1 -> Product/1
  Sum1/1 -> Mux3/1
  Mux3/1 -> R(theta)*p/1
  Product/1 -> Demux/1
  Product1/1 -> Demux1/1
  Demux/1 -> Sum1/1
  Demux1/2 -> Sum1/2
  Demux1/1 -> Sum2/2
  Demux/2 -> Sum2/1

== system Drone_BBall_Developer/EMP Mechanics//Dynamics/EMP Dynamics 1/Rotation Matrx1 ==
  p : Inport
  theta : Inport  Port=2
  Cos : Trigonometry  Operator=cos
  Demux : Demux  Outputs=2
  Demux1 : Demux  Outputs=2
  Mux3 : Mux  Inputs=2
  Product : Product
  Product1 : Product
  Sin : Trigonometry
  Sum1 : Sum
  Sum2 : Sum  Inputs=+-
  R(theta)*p : Outport  VectorParamsAs1DForOutWhenUnconnected=off
  wires:
  p/1 -> Product/2, Product1/2
  Sum2/1 -> Mux3/2
  Sin/1 -> Product1/1
  theta/1 -> Cos/1, Sin/1
  Cos/1 -> Product/1
  Sum1/1 -> Mux3/1
  Mux3/1 -> R(theta)*p/1
  Product/1 -> Demux/1
  Product1/1 -> Demux1/1
  Demux/1 -> Sum1/1
  Demux1/2 -> Sum1/2
  Demux1/1 -> Sum2/2
  Demux/2 -> Sum2/1

== system Drone_BBall_Developer/EMP Mechanics//Dynamics/EMP Dynamics 2/Rotation Matrx ==
  p : Inport
  theta : Inport  Port=2
  Cos : Trigonometry  Operator=cos
  Demux : Demux  Outputs=2
  Demux1 : Demux  Outputs=2
  Mux3 : Mux  Inputs=2
  Product : Product
  Product1 : Product
  Sin : Trigonometry
  Sum1 : Sum
  Sum2 : Sum  Inputs=+-
  R(theta)*p : Outport  VectorParamsAs1DForOutWhenUnconnected=off
  wires:
  p/1 -> Product/2, Product1/2
  Sum2/1 -> Mux3/2
  Sin/1 -> Product1/1
  theta/1 -> Cos/1, Sin/1
  Cos/1 -> Product/1
  Sum1/1 -> Mux3/1
  Mux3/1 -> R(theta)*p/1
  Product/1 -> Demux/1
  Product1/1 -> Demux1/1
  Demux/1 -> Sum1/1
  Demux1/2 -> Sum1/2
  Demux1/1 -> Sum2/2
  Demux/2 -> Sum2/1

== system Drone_BBall_Developer/EMP Mechanics//Dynamics/EMP Dynamics 2/Rotation Matrx1 ==
  p : Inport
  theta : Inport  Port=2
  Cos : Trigonometry  Operator=cos
  Demux : Demux  Outputs=2
  Demux1 : Demux  Outputs=2
  Mux3 : Mux  Inputs=2
  Product : Product
  Product1 : Product
  Sin : Trigonometry
  Sum1 : Sum
  Sum2 : Sum  Inputs=+-
  R(theta)*p : Outport  VectorParamsAs1DForOutWhenUnconnected=off
  wires:
  p/1 -> Product/2, Product1/2
  Sum2/1 -> Mux3/2
  Sin/1 -> Product1/1
  theta/1 -> Cos/1, Sin/1
  Cos/1 -> Product/1
  Sum1/1 -> Mux3/1
  Mux3/1 -> R(theta)*p/1
  Product/1 -> Demux/1
  Product1/1 -> Demux1/1
  Demux/1 -> Sum1/1
  Demux1/2 -> Sum1/2
  Demux1/1 -> Sum2/2
  Demux/2 -> Sum2/1

== system Drone_BBall_Developer/Drone 1 Controller/Quadcopter Dynamical Controller/Diff btwn Angles/Wrap Angle ==
  raw : Inport
  Gain : Gain  Gain=2
  Mod : Math  Operator=mod  SignedPower=on  SaturateOnIntegerOverflow=on
  Pi : Constant  Value=pi  OutDataTypeStr=Inherit: Inherit via back propagation
  Sum3 : Sum  Inputs=|+-
  Sum4 : Sum  Inputs=|++
  wrap : Outport  VectorParamsAs1DForOutWhenUnconnected=off
  wires:
  Sum4/1 -> Mod/1
  Pi/1 -> Sum4/2, Sum3/2, Gain/1
  Sum3/1 -> wrap/1
  raw/1 -> Sum4/1
  Mod/1 -> Sum3/1
  Gain/1 -> Mod/2

== system Drone_BBall_Developer/Drone 1 Controller/Quadcopter Dynamical Controller (Arena Frame)/Diff btwn Angles/Wrap Angle ==
  raw : Inport
  Gain : Gain  Gain=2
  Mod : Math  Operator=mod  SignedPower=on  SaturateOnIntegerOverflow=on
  Pi : Constant  Value=pi  OutDataTypeStr=Inherit: Inherit via back propagation
  Sum3 : Sum  Inputs=|+-
  Sum4 : Sum  Inputs=|++
  wrap : Outport  VectorParamsAs1DForOutWhenUnconnected=off
  wires:
  Sum4/1 -> Mod/1
  Pi/1 -> Sum4/2, Sum3/2, Gain/1
  Sum3/1 -> wrap/1
  raw/1 -> Sum4/1
  Mod/1 -> Sum3/1
  Gain/1 -> Mod/2

== system Drone_BBall_Developer/Drone 1 Controller/Quadcopter Dynamical Controller (Drone Frame)/Diff btwn Angles/Wrap Angle ==
  raw : Inport
  Gain : Gain  Gain=2
  Mod : Math  Operator=mod  SignedPower=on  SaturateOnIntegerOverflow=on
  Pi : Constant  Value=pi  OutDataTypeStr=Inherit: Inherit via back propagation
  Sum3 : Sum  Inputs=|+-
  Sum4 : Sum  Inputs=|++
  wrap : Outport  VectorParamsAs1DForOutWhenUnconnected=off
  wires:
  Sum4/1 -> Mod/1
  Pi/1 -> Sum4/2, Sum3/2, Gain/1
  Sum3/1 -> wrap/1
  raw/1 -> Sum4/1
  Mod/1 -> Sum3/1
  Gain/1 -> Mod/2

== system Drone_BBall_Developer/Drone 1 Dynamics/Hook Plant/Tether Dynamics/Rotation Matrix CW ==
  p : Inport
  theta : Inport  Port=2
  Cos : Trigonometry  Operator=cos
  Demux : Demux  Outputs=2
  Demux1 : Demux  Outputs=2
  Mux3 : Mux  Inputs=2
  Product : Product
  Product1 : Product
  Sin : Trigonometry
  Sum1 : Sum
  Sum2 : Sum  Inputs=+-
  R(theta)*p : Outport  VectorParamsAs1DForOutWhenUnconnected=off
  wires:
  p/1 -> Product/2, Product1/2
  Sum2/1 -> Mux3/2
  Sin/1 -> Product1/1
  theta/1 -> Cos/1, Sin/1
  Cos/1 -> Product/1
  Sum1/1 -> Mux3/1
  Mux3/1 -> R(theta)*p/1
  Product/1 -> Demux/1
  Product1/1 -> Demux1/1
  Demux/1 -> Sum1/1
  Demux1/2 -> Sum1/2
  Demux1/1 -> Sum2/2
  Demux/2 -> Sum2/1

== system Drone_BBall_Developer/Drone 1 Dynamics/Quadcopter Plant/Rotational Dynamics/Wrap Angle ==
  raw : Inport
  Gain : Gain  Gain=2
  Mod : Math  Operator=mod  SignedPower=on  SaturateOnIntegerOverflow=on
  Pi : Constant  Value=pi  OutDataTypeStr=Inherit: Inherit via back propagation
  Sum3 : Sum  Inputs=|+-
  Sum4 : Sum  Inputs=|++
  wrap : Outport  VectorParamsAs1DForOutWhenUnconnected=off
  wires:
  Sum4/1 -> Mod/1
  Pi/1 -> Sum4/2, Sum3/2, Gain/1
  Sum3/1 -> wrap/1
  raw/1 -> Sum4/1
  Mod/1 -> Sum3/1
  Gain/1 -> Mod/2

== system Drone_BBall_Developer/Drone 2 Dynamics/Hook Plant/Tether Dynamics/Rotation Matrix CW ==
  p : Inport
  theta : Inport  Port=2
  Cos : Trigonometry  Operator=cos
  Demux : Demux  Outputs=2
  Demux1 : Demux  Outputs=2
  Mux3 : Mux  Inputs=2
  Product : Product
  Product1 : Product
  Sin : Trigonometry
  Sum1 : Sum
  Sum2 : Sum  Inputs=+-
  R(theta)*p : Outport  VectorParamsAs1DForOutWhenUnconnected=off
  wires:
  p/1 -> Product/2, Product1/2
  Sum2/1 -> Mux3/2
  Sin/1 -> Product1/1
  theta/1 -> Cos/1, Sin/1
  Cos/1 -> Product/1
  Sum1/1 -> Mux3/1
  Mux3/1 -> R(theta)*p/1
  Product/1 -> Demux/1
  Product1/1 -> Demux1/1
  Demux/1 -> Sum1/1
  Demux1/2 -> Sum1/2
  Demux1/1 -> Sum2/2
  Demux/2 -> Sum2/1

== system Drone_BBall_Developer/Drone 2 Dynamics/Quadcopter Plant/Rotational Dynamics/Wrap Angle ==
  raw : Inport
  Gain : Gain  Gain=2
  Mod : Math  Operator=mod  SignedPower=on  SaturateOnIntegerOverflow=on
  Pi : Constant  Value=pi  OutDataTypeStr=Inherit: Inherit via back propagation
  Sum3 : Sum  Inputs=|+-
  Sum4 : Sum  Inputs=|++
  wrap : Outport  VectorParamsAs1DForOutWhenUnconnected=off
  wires:
  Sum4/1 -> Mod/1
  Pi/1 -> Sum4/2, Sum3/2, Gain/1
  Sum3/1 -> wrap/1
  raw/1 -> Sum4/1
  Mod/1 -> Sum3/1
  Gain/1 -> Mod/2

== matlab function Drone_BBall_Developer/Drone 1 Controller/Magnet Controller ==
  data: X_ball input; mag_on output; t input; t_hold_prev input; t_hold output
function [mag_on,t_hold] = fcn(X_ball,t,t_hold_prev)

% OUTPUTS
% mag_on: 1 = magnet activated; 0 = magnet deactivated
% t_hold: time when the magnet will be reactivated

% INPUTS
% X_ball: [6x1] state of ball
% t: simulation time
% t_hold_prev: output from previous time this function ran

hoop_position = [8; 8.5]; % define the center of the hoop
relative_ball_position  = X_ball([1 3]) - hoop_position;
ball_velocity = X_ball([2 4]);

t_hold = t_hold_prev; % keep track of when to reactivate the magnet

mag_on = 1; % assume the magnet should be on

% if relative_ball_position(2) > 1 % if the ball is 1m above the hoop
%     if abs(relative_ball_position(1)) < 1 % and centered above it
%         if abs(ball_velocity(1)) < 1 % and if the ball's horizontal speed is low
%             mag_on = 0; % deactivate the magnet to release the ball
%             t_hold = t + 1.0; % and plan to reactivate the magnet in 1.0 seconds
%         end
%     end

time = (hoop_position(1) - X_ball(1)) / X_ball(2); % from (x_f - x_0) / v_0x
g = 9.81;

%if X_ball(1) < (hoop_position(1) - 4) % if the ball is behind the hoop
%if (X_ball(3) - (hoop_position(2) + (X_ball(4)*time) - (0.5*g*time*time)) > -0.1) & (X_ball(3) - (hoop_position(2) + (X_ball(4)*time) - (0.5*g*time*time)) < 0.1) % projectile motion
if abs((X_ball(3) - hoop_position(2) + (X_ball(4)*time) - (0.5*g*time*time))) < 0.1
    if abs(X_ball(2)/X_ball(4)) > 0.1
            mag_on = 0; % deactivate the magnet to release the ball
            t_hold = t + 1.0; % and plan to reactivate the magnet in 1.0 seconds
    %end
    
    elseif t < t_hold_prev % if the hold time has not yet elapsed
            mag_on = 0; % keep the magnet deactivated

    end

end

== matlab function Drone_BBall_Developer/Drone 1 Controller/Posession Detection ==
  data: X_drone input; X_ball input; possession output; F_tether input; possession_prev input
function possession = fcn(X_drone,X_ball,F_tether,possession_prev)

% OUTPUTS
% possession: 1 = have possession; 0 = don't have possession

% INPUTS
% X_drone: [6x1] state of drone
% X_ball: [6x1] state of ball
% F_tether: [2x1] force of tether, relative to drone
% possession_prev: output from previous time this function ran

relative_ball_position = X_ball([1 3]) - X_drone([1 3]);

possession = possession_prev; % start with the assumption that nothing has changed

if possession_prev % if previously had possession
    if norm(relative_ball_position) > 2.5 % and if ball is more than 2.5 m away
        possession = 0; % assume possession has been lost
    end
    
elseif norm(F_tether) > 5 % and if tether force is greater than 5 N % if didn't previously have possession
        possession = 1; % assume possession has been gained
    
elseif (X_drone(3) < 1.5) && (X_ball(3) < 1) && (X_drone(2) < 1) && (norm(F_tether) < 5) %prevents the drone from getting stuck when the ball is on the ground
    possession = 1;
    
end

%end

== matlab function Drone_BBall_Developer/Drone 1 Controller/Finite State Machine ==
  data: X_drone input; X_ball input; possession input; X_catch input; freefall input; X_d output; mag_on input; state_prev input; state output
function [X_d,state] = fcn(X_drone,X_ball,possession,X_catch,freefall,mag_on,state_prev)

% OUTPUTS
% X_d: [6x1] desired state of drone (velocities set to zero)
% state: 1 - don't have possession, try to get possession
%        2 - have possession, try to score basket
%        3 - just took a shot, wait on possible rebound

% INPUTS
% X_drone: [6x1] state of drone (not currently used, but you likely will)
% X_ball: [6x1] state of ball
% possession: 1 = have possession; 0 = don't have possession
% X_catch: [6x1] estimated state of the ball when the drone will catch it
% freefall: 1 = ball is estimated to be in freefall
% mag_on: 1 = magnet activated; 0 = magnet deactivated
% state_prev: state from previous time this function ran

% NOTE: the initial state is set in the memory block below this fcn block

g = 9.81;
r_ball = 0.3;
ball_velocity = X_ball([2 4]);


relative_hook_position = [0;0;-1.5;0;0;0]; % position of hook relative to drone

state = state_prev; % assume state will not change

X_d = X_drone; % if state doesn't specify, maintain current position

if state_prev == 1 % don't have possession, try to get possession
        
    if freefall % i.e., ball is free, fly to estimated intercept point
        X_d = X_catch - relative_hook_position;
    elseif (X_ball(3) < 1)
        %X_d = X_ball - relative_hook_position;
        X_d(3) = X_ball(3) - relative_hook_position(3);
        X_d(1) = X_ball(1);

    end
    
    if possession % if gain possession
        state = 2; % try to score basket
        
    end
    
elseif state_prev == 2 % have possession, try to score basket
    X_d = [8;0;13;0;0;0]; % try to take a shot 2 m above the hoop
    
%     if (X_ball(3) < 2) && (X_ball(4) < 1) && (X_ball(2) < 1) % if the ball is on the ground
%         X_d = [8;0;13;0;0;0]; % try to take a shot 2 m above the hoop
%     end
    
    if mag_on == 0 % if have taken a shot
        state = 3; % wait for possible rebound
    elseif possession == 0 % otherwise, if lose possession
        state = 1; % try to regain possession
    end
    
elseif state_prev == 3 % just took a shot, wait on possible rebound
    X_d = X_catch; % hold position 2 m above the hoop
    if mag_on % wait for the magnet to reactivate
        state = 1; % try to regain possession (ball may have reset)
    end
       
end

end

== matlab function Drone_BBall_Developer/Drone 1 Controller/EMP Controller ==
  data: X_drone input; fire_emp output; X_opponent input; emp_armed input
function fire_emp  = fcn(X_drone,X_opponent,emp_armed)

% OUTPUTS
% fire_emp: 1 = fire EMP; 0 = don't fire EMP

% INPUTS
% X_drone: [6x1] state of drone
% X_opponent: [6x1] state of opponent
% emp_armed: 1 = EMP ready to fire; 0 = EMP recharging

rel_opp_pos = X_opponent - X_drone; % relative opponent position
rel_opp_angle = -(pi/2 + atan2(rel_opp_pos(3),rel_opp_pos(1))); % angle to opponent

fire_emp = 0; % assume EMP will not be fired

if emp_armed % if EMP is ready to fire
    if abs(rel_opp_angle - X_drone(5)) < (10 * pi/180) % and if EMP is aimed within 10 degrees of opponent
        fire_emp = 1; % fire EMP (note that emp_fire must be set to zero to rearm EMP)
    end
end

end

== matlab function Drone_BBall_Developer/Drone 1 Controller/Flipover Decector ==
  data: X_drone input; flip output; flip_prev input
function flip = fcn(X_drone,flip_prev)

% OUTPUTS
% flip: 1 = execute flipover; 0 = fly normallly

% INPUTS
% X_drone: [6x1] state of drone
% flip_prev: output from previous time this function ran

flip = flip_prev; % assume continue previous behavior

if flip_prev % if already executing a flipover
    if abs(X_drone(5)) < (90 * pi/180) % if upright again
        flip = 0; % stop flipover execution
    end
else
    if abs(X_drone(5)) > (170 * pi/180) % if upsidedown
        if X_drone(3) < 0.5 % and if less than 0.5 m above ground
            flip = 1; % begin executing flip
        end
    end
end

end
